simulink model "ros2webots_go_to_point_controller_model_cg"  (R2023a)
settings: Solver=FixedStepDiscrete  StartTime=0.0  StopTime=inf  FixedStep=0.05  RelTol=1e-3  EnableMultiTasking=on
model workspace (MAT data in the model file):
  Logfile_Data_Object = robotics.ros.BagSelection
  Logfile_Data_Object.FilePath = '\\wsl.localhost\ubuntu\home\mjavadzallaghi\ros2_ws\ros2webots\baglog\rosbot_data_20240125_225927.bag'
  Logfile_Data_Object.StartTime = 1706210981.23
  Logfile_Data_Object.EndTime = 1706211126.25
  Logfile_Data_Object.NumMessages = 508
  Logfile_Data_Object.AvailableTopics = table
  Logfile_Data_Object.AvailableTopics.data{1} = [73; 435]
  Logfile_Data_Object.AvailableTopics.data{2} = categorical
  Logfile_Data_Object.AvailableTopics.data{2}.categoryNames = {'geometry_msgs/Twist'; 'sensor_msgs/Imu'}
  Logfile_Data_Object.AvailableTopics.data{2}.codes = [1; 2]
  Logfile_Data_Object.AvailableTopics.data{3}{1} = 'geometry_msgs/Vector3 Linear
    |   double X
    |   double Y
    |   double Z
    | geometry_msgs/Vector3 Angular
    |   double X
    |   double Y
    |   double Z
    | '
  Logfile_Data_Object.AvailableTopics.data{3}{2} = 'std_msgs/Header Header
    |   uint32 Seq
    |   Time Stamp
    |   char FrameId
    | geometry_msgs/Quaternion Orientation
    |   double X
    |   double Y
    |   double Z
    |   double W
    | double[9] OrientationCovariance
    | geometry_msgs/Vector3 AngularVelocity
    |   double X
    |   double Y
    |   double Z
    | double[9] AngularVelocityCovariance
    | geometry_msgs/Vector3 LinearAcceleration
    |   double X
    |   double Y
    |   double Z
    | double[9] LinearAccelerationCovariance
    | '
  Logfile_Data_Object.AvailableTopics.ndims = 2
  Logfile_Data_Object.AvailableTopics.nrows = 2
  Logfile_Data_Object.AvailableTopics.rownames = {'/webots/rosbot/command_vel'; '/webots/rosbot/imu'}
  Logfile_Data_Object.AvailableTopics.nvars = 3
  Logfile_Data_Object.AvailableTopics.varnames = {'NumMessages', 'MessageType', 'MessageDefinition'}
  Logfile_Data_Object.AvailableTopics.props.useVariableNamesOriginal = 0
  Logfile_Data_Object.AvailableTopics.props.useDimensionNamesOriginal = 0
  Logfile_Data_Object.AvailableTopics.props.CustomProps = struct()
  Logfile_Data_Object.AvailableTopics.props.VariableCustomProps = struct()
  Logfile_Data_Object.AvailableTopics.props.versionSavedFrom = 4
  Logfile_Data_Object.AvailableTopics.props.minCompatibleVersion = 1
  Logfile_Data_Object.AvailableTopics.props.incompatibilityMsg = ''
  Logfile_Data_Object.AvailableTopics.props.VersionSavedFrom = 4
  Logfile_Data_Object.AvailableTopics.props.Description = ''
  Logfile_Data_Object.AvailableTopics.props.VariableNamesOriginal = {}
  Logfile_Data_Object.AvailableTopics.props.DimensionNames = {'Row', 'Variables'}
  Logfile_Data_Object.AvailableTopics.props.DimensionNamesOriginal = {}
  Logfile_Data_Object.AvailableTopics.props.UserData = []
  Logfile_Data_Object.AvailableTopics.props.VariableDescriptions = {}
  Logfile_Data_Object.AvailableTopics.props.VariableUnits = {}
  Logfile_Data_Object.AvailableTopics.props.VariableContinuity = {}
  Logfile_Data_Object.MessageList = table
  Logfile_Data_Object.MessageList.data{1} = [1706210981.23 1706210981.23 1706210981.23 1706210983.05 1706210983.38 1706210983.7 1706210984.04 1706210984.38 1706210984.72 1706210985.07 1706210985.41 1706210985.73 ... (508 elements, 508x1)]
  Logfile_Data_Object.MessageList.data{2} = categorical
  Logfile_Data_Object.MessageList.data{2}.categoryNames = {'/webots/rosbot/command_vel'; '/webots/rosbot/imu'}
  Logfile_Data_Object.MessageList.data{2}.codes = [1; 1; 1; 2; 2; 2; 2; 2; 2; 2; 2; 1; 1; 1; 2; 2; 2; 2; 2; 2; 2; 2; 2; 2; 2; 2; 2; 2; 2; 2; 2; 2; 2; 2; 2; 2; 2; 2; 1; 1; 1; 2; 2; 2; 2; 2; 2; 2; 2; 2; 2; 2; 2; 2; 2; 2; 2; 2; 2; 2; 2; 2; 2; 2; 2; 2; 2; 1; 1; 1; 2; 2; 2; 2; 2; 2; 2; 2; 2; 2; 2; 2; 2; 2; 2; 2; 2; 2; 2; 2; 2; 1; 1; 1; 2; 2; 2; 2; 2; 2; 2; 2; 2; 2; 2; 2; 2; 2; 2; 2; 2; 2; 2; 2; 2; 2; 2; 2; 1; 1; 2; 1; 2; 2; 2; 2; 2; 2; 2; 2; 2; 2; 2; 2; 2; 2; 2; 2; 2; 2; 2; 2; 2; 2; 2; 2; 2; 2; 2; 2; 2; 2; 2; 2; 2; 2; 2; 2; 2; 2; 2; 2; 2; 2; 2; 2; 1; 1; 1; 2; 2; 2; 2; 2; 2; 2; 2; 2; 2; 2; 2; 2; 2; 2; 2; 2; 2; 2; 2; 2; 2; 2; 2; 1; 1; 1; 2; 2; 2; 2; 2; 2; 2; 2; 2; 2; 2; 2; 2; 2; 2; 2; 2; 2; 2; 2; 2; 2; 2; 2; 2; 2; 2; 1; 1; 1; 2; 2; 2; 2; 2; 2; 2; 2; 2; 2; 2; 2; 2; 2; 2; 2; 2; 2; 2; 2; 2; 2; 2; 2; 2; 2; 1; 1; 1; 2; 2; 2; 2; 2; 2; 2; 2; 2; 2; 2; 2; 2; 2; 2; 2; 2; 2; 2; 2; 1; 1; 1; 2; 2; 2; 2; 2; 2; 2; 2; 2; 2; 2; 2; 2; 2; 2; 2; 2; 2; 2; 2; 2; 2; 2; 2; 2; 1; 1; 1; 2; 2; 2; 2; 2; 2; 2; 1; 1; 2; 1; 2; 2; 2; 2; 2; 2; 1; 1; 1; 2; 2; 2; 2; 2; 2; 2; 2; 2; 2; 2; 2; 1; 1; 1; 2; 2; 2; 2; 2; 2; 2; 2; 2; 2; 2; 2; 2; 2; 2; 2; 2; 2; 2; 1; 1; 1; 2; 2; 2; 2; 2; 2; 2; 2; 2; 1; 1; 1; 2; 2; 2; 2; 2; 2; 2; 2; 2; 2; 2; 2; 1; 1; 1; 2; 2; 2; 2; 2; 2; 1; 1; 1; 2; 2; 2; 2; 2; 2; 2; 2; 2; 2; 2; 2; 1; 1; 1; 2; 2; 2; 2; 2; 2; 2; 2; 2; 2; 1; 1; 1; 2; 2; 2; 2; 2; 2; 2; 2; 2; 2; 1; 1; 1; 2; 2; 2; 2; 2; 2; 2; 1; 1; 1; 2; 2; 2; 2; 2; 2; 2; 2; 2; 2; 2; 2; 2; 2; 2; 2; 1; 1; 1; 2; 2; 2; 2; 2; 2; 2; 2; 2; 2; 2; 2; 2; 2; 2; 2; 1; 2; 2; 2; 2; 2; 2; 2; 2; 2; 2; 2; 2; 2; 2; 2; 2; 2; 2; 2; 2; 2; 2]
  Logfile_Data_Object.MessageList.data{3} = categorical
  Logfile_Data_Object.MessageList.data{3}.categoryNames = {'geometry_msgs/Twist'; 'sensor_msgs/Imu'}
  Logfile_Data_Object.MessageList.data{3}.codes = [1; 1; 1; 2; 2; 2; 2; 2; 2; 2; 2; 1; 1; 1; 2; 2; 2; 2; 2; 2; 2; 2; 2; 2; 2; 2; 2; 2; 2; 2; 2; 2; 2; 2; 2; 2; 2; 2; 1; 1; 1; 2; 2; 2; 2; 2; 2; 2; 2; 2; 2; 2; 2; 2; 2; 2; 2; 2; 2; 2; 2; 2; 2; 2; 2; 2; 2; 1; 1; 1; 2; 2; 2; 2; 2; 2; 2; 2; 2; 2; 2; 2; 2; 2; 2; 2; 2; 2; 2; 2; 2; 1; 1; 1; 2; 2; 2; 2; 2; 2; 2; 2; 2; 2; 2; 2; 2; 2; 2; 2; 2; 2; 2; 2; 2; 2; 2; 2; 1; 1; 2; 1; 2; 2; 2; 2; 2; 2; 2; 2; 2; 2; 2; 2; 2; 2; 2; 2; 2; 2; 2; 2; 2; 2; 2; 2; 2; 2; 2; 2; 2; 2; 2; 2; 2; 2; 2; 2; 2; 2; 2; 2; 2; 2; 2; 2; 1; 1; 1; 2; 2; 2; 2; 2; 2; 2; 2; 2; 2; 2; 2; 2; 2; 2; 2; 2; 2; 2; 2; 2; 2; 2; 2; 1; 1; 1; 2; 2; 2; 2; 2; 2; 2; 2; 2; 2; 2; 2; 2; 2; 2; 2; 2; 2; 2; 2; 2; 2; 2; 2; 2; 2; 2; 1; 1; 1; 2; 2; 2; 2; 2; 2; 2; 2; 2; 2; 2; 2; 2; 2; 2; 2; 2; 2; 2; 2; 2; 2; 2; 2; 2; 2; 1; 1; 1; 2; 2; 2; 2; 2; 2; 2; 2; 2; 2; 2; 2; 2; 2; 2; 2; 2; 2; 2; 2; 1; 1; 1; 2; 2; 2; 2; 2; 2; 2; 2; 2; 2; 2; 2; 2; 2; 2; 2; 2; 2; 2; 2; 2; 2; 2; 2; 2; 1; 1; 1; 2; 2; 2; 2; 2; 2; 2; 1; 1; 2; 1; 2; 2; 2; 2; 2; 2; 1; 1; 1; 2; 2; 2; 2; 2; 2; 2; 2; 2; 2; 2; 2; 1; 1; 1; 2; 2; 2; 2; 2; 2; 2; 2; 2; 2; 2; 2; 2; 2; 2; 2; 2; 2; 2; 1; 1; 1; 2; 2; 2; 2; 2; 2; 2; 2; 2; 1; 1; 1; 2; 2; 2; 2; 2; 2; 2; 2; 2; 2; 2; 2; 1; 1; 1; 2; 2; 2; 2; 2; 2; 1; 1; 1; 2; 2; 2; 2; 2; 2; 2; 2; 2; 2; 2; 2; 1; 1; 1; 2; 2; 2; 2; 2; 2; 2; 2; 2; 2; 1; 1; 1; 2; 2; 2; 2; 2; 2; 2; 2; 2; 2; 1; 1; 1; 2; 2; 2; 2; 2; 2; 2; 1; 1; 1; 2; 2; 2; 2; 2; 2; 2; 2; 2; 2; 2; 2; 2; 2; 2; 2; 1; 1; 1; 2; 2; 2; 2; 2; 2; 2; 2; 2; 2; 2; 2; 2; 2; 2; 2; 1; 2; 2; 2; 2; 2; 2; 2; 2; 2; 2; 2; 2; 2; 2; 2; 2; 2; 2; 2; 2; 2; 2]
  Logfile_Data_Object.MessageList.data{4} = [5438 5532 5626 5720 6078 6436 6794 7152 7510 7868 8226 8584 ... (508 elements, 508x1)]
  Logfile_Data_Object.MessageList.ndims = 2
  Logfile_Data_Object.MessageList.nrows = 508
  Logfile_Data_Object.MessageList.nvars = 4
  Logfile_Data_Object.MessageList.varnames = {'Time', 'Topic', 'MessageType', 'FileOffset'}
  Logfile_Data_Object.MessageList.props.useVariableNamesOriginal = 0
  Logfile_Data_Object.MessageList.props.useDimensionNamesOriginal = 0
  Logfile_Data_Object.MessageList.props.CustomProps = struct()
  Logfile_Data_Object.MessageList.props.VariableCustomProps = struct()
  Logfile_Data_Object.MessageList.props.versionSavedFrom = 4
  Logfile_Data_Object.MessageList.props.minCompatibleVersion = 1
  Logfile_Data_Object.MessageList.props.incompatibilityMsg = ''
  Logfile_Data_Object.MessageList.props.VersionSavedFrom = 4
  Logfile_Data_Object.MessageList.props.Description = ''
  Logfile_Data_Object.MessageList.props.VariableNamesOriginal = {}
  Logfile_Data_Object.MessageList.props.DimensionNames = {'Row', 'Variables'}
  Logfile_Data_Object.MessageList.props.DimensionNamesOriginal = {}
  Logfile_Data_Object.MessageList.props.UserData = []
  Logfile_Data_Object.MessageList.props.VariableDescriptions = {}
  Logfile_Data_Object.MessageList.props.VariableUnits = {}
  Logfile_Data_Object.MessageList.props.VariableContinuity = {}
  Logfile_Data_Object.RawMessageBuffer = containers.Map
  Logfile_Data_Object.RawMessageBuffer.serialization.keys = {}
  Logfile_Data_Object.RawMessageBuffer.serialization.values = {}
  Logfile_Data_Object.RawMessageBuffer.serialization.uniformity = 0
  Logfile_Data_Object.RawMessageBuffer.serialization.keyType = 'char'
  Logfile_Data_Object.RawMessageBuffer.serialization.valueType = 'any'
  Logfile_Data_Object.ImgMessageBuffer = containers.Map
  Logfile_Data_Object.ImgMessageBuffer.serialization.keys = {}
  Logfile_Data_Object.ImgMessageBuffer.serialization.values = {}
  Logfile_Data_Object.ImgMessageBuffer.serialization.uniformity = 0
  Logfile_Data_Object.ImgMessageBuffer.serialization.keyType = 'char'
  Logfile_Data_Object.ImgMessageBuffer.serialization.valueType = 'any'
  Logfile_Data_Object.PointCloudBuffer = containers.Map
  Logfile_Data_Object.PointCloudBuffer.serialization.keys = {}
  Logfile_Data_Object.PointCloudBuffer.serialization.values = {}
  Logfile_Data_Object.PointCloudBuffer.serialization.uniformity = 0
  Logfile_Data_Object.PointCloudBuffer.serialization.keyType = 'char'
  Logfile_Data_Object.PointCloudBuffer.serialization.valueType = 'any'
  Logfile_Data_Object.LaserScanBuffer = containers.Map
  Logfile_Data_Object.LaserScanBuffer.serialization.keys = {}
  Logfile_Data_Object.LaserScanBuffer.serialization.values = {}
  Logfile_Data_Object.LaserScanBuffer.serialization.uniformity = 0
  Logfile_Data_Object.LaserScanBuffer.serialization.keyType = 'char'
  Logfile_Data_Object.LaserScanBuffer.serialization.valueType = 'any'
  Logfile_Data_Object.TopicTypeMap = containers.Map
  Logfile_Data_Object.TopicTypeMap.serialization.keys = {'/webots/rosbot/command_vel', '/webots/rosbot/imu'}
  Logfile_Data_Object.TopicTypeMap.serialization.values = {'geometry_msgs/Twist', 'sensor_msgs/Imu'}
  Logfile_Data_Object.TopicTypeMap.serialization.uniformity = 1
  Logfile_Data_Object.TopicTypeMap.serialization.keyType = 'char'
  Logfile_Data_Object.TopicTypeMap.serialization.valueType = 'char'
  Logfile_Data_Object.TopicDefinitionMap = containers.Map
  Logfile_Data_Object.TopicDefinitionMap.serialization.keys = {'/webots/rosbot/command_vel', '/webots/rosbot/imu'}
  Logfile_Data_Object.TopicDefinitionMap.serialization.values{1} = 'geometry_msgs/Vector3 Linear
    |   double X
    |   double Y
    |   double Z
    | geometry_msgs/Vector3 Angular
    |   double X
    |   double Y
    |   double Z
    | '
  Logfile_Data_Object.TopicDefinitionMap.serialization.values{2} = 'std_msgs/Header Header
    |   uint32 Seq
    |   Time Stamp
    |   char FrameId
    | geometry_msgs/Quaternion Orientation
    |   double X
    |   double Y
    |   double Z
    |   double W
    | double[9] OrientationCovariance
    | geometry_msgs/Vector3 AngularVelocity
    |   double X
    |   double Y
    |   double Z
    | double[9] AngularVelocityCovariance
    | geometry_msgs/Vector3 LinearAcceleration
    |   double X
    |   double Y
    |   double Z
    | double[9] LinearAccelerationCovariance
    | '
  Logfile_Data_Object.TopicDefinitionMap.serialization.uniformity = 1
  Logfile_Data_Object.TopicDefinitionMap.serialization.keyType = 'char'
  Logfile_Data_Object.TopicDefinitionMap.serialization.valueType = 'char'
  Logfile_Data_Object.messageTypeMap = containers.Map
  Logfile_Data_Object.messageTypeMap.serialization.keys = {}
  Logfile_Data_Object.messageTypeMap.serialization.values = {}
  Logfile_Data_Object.messageTypeMap.serialization.uniformity = 0
  Logfile_Data_Object.messageTypeMap.serialization.keyType = 'char'
  Logfile_Data_Object.messageTypeMap.serialization.valueType = 'any'
  Logfile_Data_Object.Parser = robotics.ros.internal.tf.TransformationTreeParser
  Logfile_Data_Object.Parser.UseObjectMsg = 1
  Logfile_Path = '\\wsl.localhost\ubuntu\home\mjavadzallaghi\ros2_ws\ros2webots\baglog\rosbot_data_20240125_225927.bag'
  Logfile_Playback_Duration = nan
  Logfile_Playback_Offset = nan
values from neighbouring files (symbols this model uses):
  laterl_PID_kd = 0.0    [ros2webots_go_to_point_controller_model_cg.sldd]
  laterl_PID_ki = 0.2    [ros2webots_go_to_point_controller_model_cg.sldd]
  laterl_PID_kp = 1.0    [ros2webots_go_to_point_controller_model_cg.sldd]
  longitudinal_speed_gain = 0.2    [ros2webots_go_to_point_controller_model_cg.sldd]
libraries: slpidlib x2, robotmobilelib x1, SignalEditorBlockLib x1
settings Model: DataDictionary=ros2webots_go_to_point_controller_model_cg.sldd  Creator=MJava  LastModifiedBy=MJava
settings SolverCC: AllowMultiTaskInputOutput=on  AutoInsertRateTranBlk=on
settings OptimizationCC: DefaultParameterBehavior=Inlined  EnhancedBackFolding=on  PassReuseOutputArgsAs=Individual arguments  ZeroExternalMemoryAtStartup=off  ZeroInternalMemoryAtStartup=off  MaxStackSize=64  OptimizeBlockOrder=speed  DifferentSizesBufferReuse=on  OptimizationCustomize=off  EfficientTunableParamExpr=on
settings DebuggingCC: ParameterTunabilityLossMsg=error
settings SFSimCC: MATLABDynamicMemAlloc=off  SimTargetLang=C++
settings RTWCC: Description=Embedded Coder  SystemTargetFile=ert.tlc  TemplateMakefile=ert_default_tmf  GenerateReport=on  Toolchain=Microsoft Visual C++ 2019 v16.0 | nmake (64-bit Windows)  BuildConfiguration=Faster Runs  LaunchReport=on  TargetLang=C++  GenerateWebview=on  GenerateCodeMetricsReport=on  CheckMdlBeforeBuild=Warning
settings CodeAppCC: ForceParamTrailComments=on  IgnoreCustomStorageClasses=off  OperatorAnnotations=on  SimulinkDataObjDesc=on  SFDataObjDesc=on  InsertBlockDesc=on
settings ERTTargetCC: TargetLangStandard=C++11 (ISO)  CodeInterfacePackaging=C++ class  RootIOFormat=Structure reference  ERTCustomFileTemplate=example_file_process.tlc

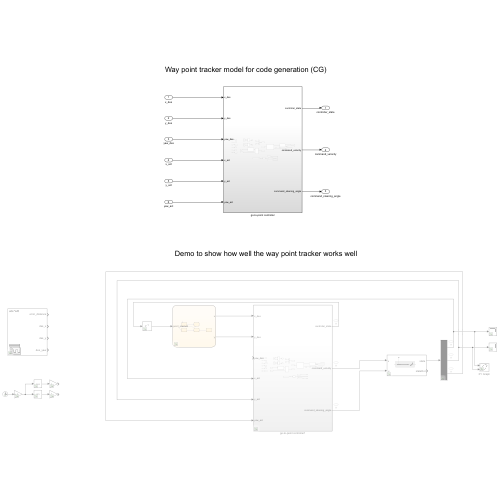
[thumbnail: Simulink's stored preview of the top-level diagram]
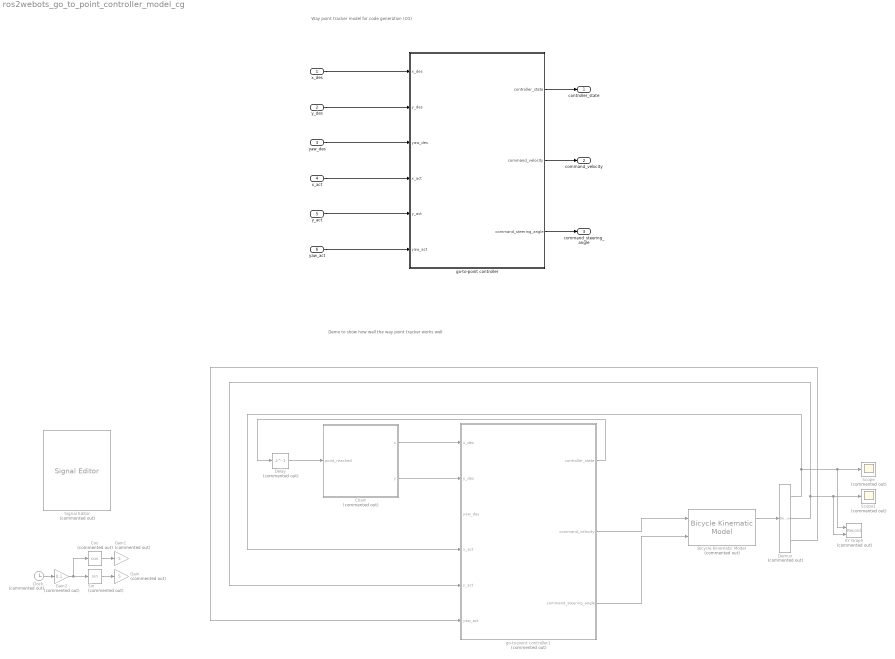
== system ros2webots_go_to_point_controller_model_cg ==
  note: Demo to show how well the way point tracker works well
  note: Way point tracker model for code generation (CG)
  x_des : Inport  OutDataTypeStr=double  PortDimensions=1
  y_des : Inport  Port=2
  yaw_des : Inport  Port=3
  x_act : Inport  Port=4
  y_act : Inport  Port=5
  yaw_act : Inport  Port=6
  Bicycle Kinematic Model : robotmobilelib/Bicycle Kinematic Model  Commented=on  VehicleInputs=Vehicle Speed & Steering Angle  WheelBase=0.2  VehicleSpeedRange=[-inf inf]  MaxSteeringAngle=pi/4  InitialState=[0; 0; 0]  SimulateUsing=Interpreted execution
  Chart : Stateflow chart  Commented=on  TreatAsAtomicUnit=on
  Clock : Clock  Commented=on
  Cos : Trigonometry  Commented=on  Operator=cos
  Delay : Delay  Commented=on  DelayLength=1  InitialCondition=1
  Demux : Demux  Commented=on  Outputs=3
  Gain : Gain  Commented=on  Gain=5
  Gain1 : Gain  Commented=on  Gain=5
  Gain2 : Gain  Commented=on  Gain=0.1
  Scope : Scope  Commented=on
  Scope1 : Scope  Commented=on
  Signal Editor : SignalEditorBlockLib/Signal Editor  Commented=on  FileName=controller_way_point_state_flow_test_scenario.mat  ActiveScenario=Scenario  ActiveSignal=error_distance  IsBus=off  OutputBusObjectStr=Bus: BusObject  SampleTime=0.05  Interpolate=off  ZeroCross=off  OutputAfterFinalValue=Setting to zero  Unit=inherit  PreserveSignalName=on  ApplySigPropsToAllScenarios=on
  Sin : Trigonometry  Commented=on
  XY Graph : Record  Commented=on  FileSettingsInternal="{\"entries\":[{\"content\":{\"excelSettings\":{\"content\":{},\"type\":\"Streamout.ExcelSettings\"}},\"type\":\"Streamout.FileSettingStorage\",\"uuid\":\"b027da48-4c5f-40c1-b71a-aa0128182c7a\"}],\"packageUris\":[\"http://schema.mathworks.com/mf0/streamout_blocks/R2020a\"],\"version\":\"1.0\"}"  Layout=[1 1]  SignalsInternal="{\"entries\":[{\"content\":{},\"type\":\"RecordBlkView.InputSignals\",\"uuid\":\"f54d1e1f-9c18-4039-bd87-6a5f989906ef\"}],\"packageUris\":[\"http://schema.mathworks.com/mf0/streamout_blocks/R2020a\"],\"version\":\"1.0\"}"  VisualizationBindings="{\"xyplotplugin\":{\"info\":[{\"series\":[],\"subplotID\":1}]}}"  CompatibilityTag=XY
  go-to-point controller : Subsystem
  go-to-point controller1 : Subsystem  Commented=on
  controller_state : Outport  PortDimensions=1
  command_velocity : Outport  Port=2  PortDimensions=1
  command_steering_angle : Outport  Port=3  PortDimensions=1
  wires:
  x_des/1 -> go-to-point controller/1(x_des)
  go-to-point controller/1(controller_state) -> controller_state/1
  y_des/1 -> go-to-point controller/2(y_des)
  y_act/1 -> go-to-point controller/5(y_act)
  x_act/1 -> go-to-point controller/4(x_act)
  yaw_des/1 -> go-to-point controller/3(yaw_des)
  yaw_act/1 -> go-to-point controller/6(yaw_act)
  go-to-point controller/2(command_velocity) -> command_velocity/1
  go-to-point controller/3(command_steering_angle) -> command_steering_angle/1
  Bicycle Kinematic Model/1 -> Demux/1
  Demux/1 -> go-to-point controller1/4(x_act), XY Graph/1, Scope/1
  Demux/2 -> go-to-point controller1/5(y_act), XY Graph/2, Scope1/1
  Demux/3 -> go-to-point controller1/6(yaw_act)
  go-to-point controller1/2(command_velocity) -> Bicycle Kinematic Model/1
  go-to-point controller1/3(command_steering_angle) -> Bicycle Kinematic Model/2
  go-to-point controller1/1(controller_state) -> Delay/1
  Delay/1 -> Chart/1(point_reached)
  Clock/1 -> Gain2/1
  Gain2/1 -> Cos/1, Sin/1
  Cos/1 -> Gain1/1
  Sin/1 -> Gain/1
  Chart/1(x) -> go-to-point controller1/1(x_des)
  Chart/2(y) -> go-to-point controller1/2(y_des)

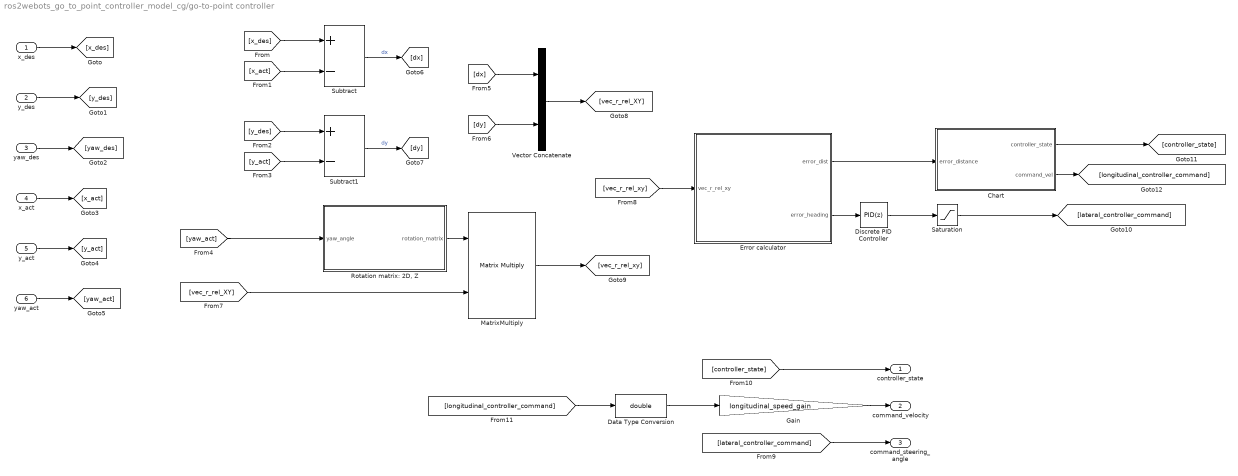
== system ros2webots_go_to_point_controller_model_cg/go-to-point controller ==
  x_des : Inport  OutDataTypeStr=double  PortDimensions=1
  y_des : Inport  Port=2  OutDataTypeStr=double  PortDimensions=1
  yaw_des : Inport  Port=3  OutDataTypeStr=double  PortDimensions=1
  x_act : Inport  Port=4  OutDataTypeStr=double  PortDimensions=1
  y_act : Inport  Port=5  OutDataTypeStr=double  PortDimensions=1
  yaw_act : Inport  Port=6  OutDataTypeStr=double  PortDimensions=1
  Chart : Stateflow chart  TreatAsAtomicUnit=on
  Data Type Conversion : DataTypeConversion  OutDataTypeStr=double  SaturateOnIntegerOverflow=off  RndMeth=Floor
  Discrete PID Controller : slpidlib/PID Controller  Controller=PID  Form=Parallel  TimeDomain=Discrete-time  UseExternalTs=off  SampleTime=-1  IntegratorMethod=Forward Euler  FilterMethod=Forward Euler  ControllerParametersSource=internal  P=laterl_PID_kp  I=laterl_PID_ki  UseKiTs=off  D=laterl_PID_kd  N=100  UseFilter=on  TunerSelectOption=Transfer Function Based (PID Tuner App)  InitialConditionSource=internal  InitialConditionForIntegrator=0  InitialConditionForFilter=0  DifferentiatorICPrevScaledInput=0  ExternalReset=none  TrackingMode=off  Kt=1  LimitOutput=off  SatLimitsSource=internal  UpperSaturationLimit=inf  LowerSaturationLimit=-inf  LinearizeAsGain=off  AntiWindupMode=none  Kb=1  LimitIntegrator=off  UpperIntegratorSaturationLimit=inf  LowerIntegratorSaturationLimit=-inf  POutMin=[]  POutMax=[]  IOutMin=[]  IOutMax=[]  DOutMin=[]  DOutMax=[]  NOutMin=[]  NOutMax=[]  SumOutMin=[]  SumOutMax=[]  SaturationOutMin=[]  SaturationOutMax=[]  PParamMin=[]  PParamMax=[]  IParamMin=[]  IParamMax=[]  DParamMin=[]  DParamMax=[]  NParamMin=[]  NParamMax=[]  KbParamMin=[]  KbParamMax=[]  KtParamMin=[]  KtParamMax=[]  KbOutMin=[]  KbOutMax=[]  KtOutMin=[]  KtOutMax=[]  IntegratorOutMin=[]  IntegratorOutMax=[]  FilterOutMin=[]  FilterOutMax=[]  SumI1OutMin=[]  SumI1OutMax=[]  SumI2OutMin=[]  SumI2OutMax=[]  SumI3OutMin=[]  SumI3OutMax=[]  SumI4OutMin=[]  SumI4OutMax=[]  SumDOutMin=[]  SumDOutMax=[]  DifferentiatorOutMin=[]  DifferentiatorOutMax=[]  FilterDiffOutCoefMin=[]  FilterDiffOutCoefMax=[]  ReciprocalOutMin=[]  ReciprocalOutMax=[]  SumDenOutMin=[]  SumDenOutMax=[]  SumNumOutMin=[]  SumNumOutMax=[]  DivideOutMin=[]  DivideOutMax=[]  UdiffTsProdOutMin=[]  UdiffTsProdOutMax=[]  NTsProdOutMin=[]  NTsProdOutMax=[]  UintegralTsProdOutMin=[]  UintegralTsProdOutMax=[]  UngainTsProdOutMin=[]  UngainTsProdOutMax=[]  ClampingZeroOutDataTypeStr=Inherit: Inherit via back propagation  ClampingZeroOutMin=[]  ClampingZeroOutMax=[]  FilterDenConstantOutDataTypeStr=Inherit: Inherit via back propagation  FilterDenConstantOutMin=[]  FilterDenConstantOutMax=[]  PCopyOutDataTypeStr=Inherit: Inherit via back propagation  PCopyOutMin=[]  PCopyOutMax=[]  NCopyOutDataTypeStr=Inherit: Inherit via back propagation  NCopyOutMin=[]  NCopyOutMax=[]  IntegratorContinuousStateAttributes=''  IntegratorStateMustResolveToSignalObject=off  IntegratorRTWStateStorageClass=Auto  FilterContinuousStateAttributes=''  FilterStateMustResolveToSignalObject=off  FilterRTWStateStorageClass=Auto  ParallelPVariant=InternalParameters  IdealPVariant=Disabled  IVariant=InternalParameters  DVariant=InternalParameters  IntegratorVariant=Discrete  SatVariant=Disabled  AWVariant=Passthrough  PCopyVariant=Disabled  TRVariant=Disabled  FdbkBlocksVariant=Forward  IdealPFdbkVariant=Disabled  SatFdbkVariant=Disabled  DerivativeFilterVariant=ForwardEulerFilter  NVariant=InternalParameters  NCopyVariant=Disabled  FilterICVariant=InternalICsFilter  IntegratorICVariant=InternalICs  ExternalResetVariant=Disabled  TRSumVariant=Passthrough  SumFdbkVariant=Disabled  SumVariant=Sum_PID  TsampFilterVariant=InternalTs  TsampNgainVariant=Passthrough  TsampIntegralVariant=Disabled_SignalSpec  ExternalSaturationOutDataTypeStr=Inherit: Same as second input
      settings: LibrarySourceBlock=simulink/Discrete/Discrete PID Controller
  Error calculator : MATLAB Function  TreatAsAtomicUnit=on
  Gain : Gain  Gain=longitudinal_speed_gain
  MatrixMultiply : Product  Multiplication=Matrix(*)
  "Rotation matrix: 2D, Z" : MATLAB Function  TreatAsAtomicUnit=on
  Saturation : Saturate  UpperLimit=pi/4  LowerLimit=-pi/4
  Subtract : Sum  Inputs=+-
  Subtract1 : Sum  Inputs=+-
  Vector Concatenate : Concatenate
  controller_state : Outport  OutDataTypeStr=uint8  PortDimensions=1
  command_velocity : Outport  Port=2  OutDataTypeStr=double  PortDimensions=1
  command_steering_angle : Outport  Port=3  OutDataTypeStr=double  PortDimensions=1
  wires:
  x_des/1 -> [x_des]
  y_des/1 -> [y_des]
  yaw_act/1 -> [yaw_act]
  y_act/1 -> [y_act]
  x_act/1 -> [x_act]
  yaw_des/1 -> [yaw_des]
  [x_des] -> Subtract/1
  [x_act] -> Subtract/2
  Subtract/1 -> [dx]  "dx"
  [y_act] -> Subtract1/2
  Subtract1/1 -> [dy]  "dy"
  [y_des] -> Subtract1/1
  "Rotation matrix: 2D, Z"/1(rotation_matrix) -> MatrixMultiply/1
  [yaw_act] -> "Rotation matrix: 2D, Z"/1(yaw_angle)
  [dx] -> Vector Concatenate/1
  [dy] -> Vector Concatenate/2
  Vector Concatenate/1 -> [vec_r_rel_XY]
  [vec_r_rel_XY] -> MatrixMultiply/2
  MatrixMultiply/1 -> [vec_r_rel_xy]
  [vec_r_rel_xy] -> Error calculator/1(vec_r_rel_xy)
  Error calculator/2(error_heading) -> Discrete PID Controller/1
  Discrete PID Controller/1 -> Saturation/1
  [lateral_controller_command] -> command_steering_angle/1
  Error calculator/1(error_dist) -> Chart/1(error_distance)
  Chart/1(controller_state) -> [controller_state]
  [controller_state] -> controller_state/1
  Chart/2(command_vel) -> [longitudinal_controller_command]
  [longitudinal_controller_command] -> Data Type Conversion/1
  Gain/1 -> command_velocity/1
  Data Type Conversion/1 -> Gain/1
  Saturation/1 -> [lateral_controller_command]

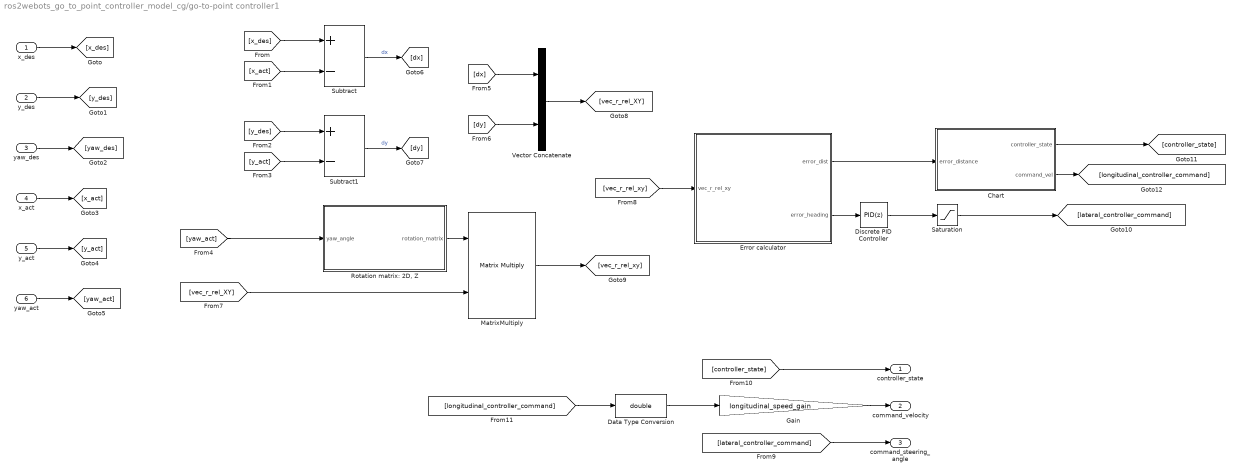
== system ros2webots_go_to_point_controller_model_cg/go-to-point controller1 ==
  x_des : Inport  OutDataTypeStr=double  PortDimensions=1
  y_des : Inport  Port=2  OutDataTypeStr=double  PortDimensions=1
  yaw_des : Inport  Port=3  OutDataTypeStr=double  PortDimensions=1
  x_act : Inport  Port=4  OutDataTypeStr=double  PortDimensions=1
  y_act : Inport  Port=5  OutDataTypeStr=double  PortDimensions=1
  yaw_act : Inport  Port=6  OutDataTypeStr=double  PortDimensions=1
  Chart : Stateflow chart  TreatAsAtomicUnit=on
  Data Type Conversion : DataTypeConversion  OutDataTypeStr=double  SaturateOnIntegerOverflow=off  RndMeth=Floor
  Discrete PID Controller : slpidlib/PID Controller  Controller=PID  Form=Parallel  TimeDomain=Discrete-time  UseExternalTs=off  SampleTime=-1  IntegratorMethod=Forward Euler  FilterMethod=Forward Euler  ControllerParametersSource=internal  P=laterl_PID_kp  I=laterl_PID_ki  UseKiTs=off  D=laterl_PID_kd  N=100  UseFilter=on  TunerSelectOption=Transfer Function Based (PID Tuner App)  InitialConditionSource=internal  InitialConditionForIntegrator=0  InitialConditionForFilter=0  DifferentiatorICPrevScaledInput=0  ExternalReset=none  TrackingMode=off  Kt=1  LimitOutput=off  SatLimitsSource=internal  UpperSaturationLimit=inf  LowerSaturationLimit=-inf  LinearizeAsGain=off  AntiWindupMode=none  Kb=1  LimitIntegrator=off  UpperIntegratorSaturationLimit=inf  LowerIntegratorSaturationLimit=-inf  POutMin=[]  POutMax=[]  IOutMin=[]  IOutMax=[]  DOutMin=[]  DOutMax=[]  NOutMin=[]  NOutMax=[]  SumOutMin=[]  SumOutMax=[]  SaturationOutMin=[]  SaturationOutMax=[]  PParamMin=[]  PParamMax=[]  IParamMin=[]  IParamMax=[]  DParamMin=[]  DParamMax=[]  NParamMin=[]  NParamMax=[]  KbParamMin=[]  KbParamMax=[]  KtParamMin=[]  KtParamMax=[]  KbOutMin=[]  KbOutMax=[]  KtOutMin=[]  KtOutMax=[]  IntegratorOutMin=[]  IntegratorOutMax=[]  FilterOutMin=[]  FilterOutMax=[]  SumI1OutMin=[]  SumI1OutMax=[]  SumI2OutMin=[]  SumI2OutMax=[]  SumI3OutMin=[]  SumI3OutMax=[]  SumI4OutMin=[]  SumI4OutMax=[]  SumDOutMin=[]  SumDOutMax=[]  DifferentiatorOutMin=[]  DifferentiatorOutMax=[]  FilterDiffOutCoefMin=[]  FilterDiffOutCoefMax=[]  ReciprocalOutMin=[]  ReciprocalOutMax=[]  SumDenOutMin=[]  SumDenOutMax=[]  SumNumOutMin=[]  SumNumOutMax=[]  DivideOutMin=[]  DivideOutMax=[]  UdiffTsProdOutMin=[]  UdiffTsProdOutMax=[]  NTsProdOutMin=[]  NTsProdOutMax=[]  UintegralTsProdOutMin=[]  UintegralTsProdOutMax=[]  UngainTsProdOutMin=[]  UngainTsProdOutMax=[]  ClampingZeroOutDataTypeStr=Inherit: Inherit via back propagation  ClampingZeroOutMin=[]  ClampingZeroOutMax=[]  FilterDenConstantOutDataTypeStr=Inherit: Inherit via back propagation  FilterDenConstantOutMin=[]  FilterDenConstantOutMax=[]  PCopyOutDataTypeStr=Inherit: Inherit via back propagation  PCopyOutMin=[]  PCopyOutMax=[]  NCopyOutDataTypeStr=Inherit: Inherit via back propagation  NCopyOutMin=[]  NCopyOutMax=[]  IntegratorContinuousStateAttributes=''  IntegratorStateMustResolveToSignalObject=off  IntegratorRTWStateStorageClass=Auto  FilterContinuousStateAttributes=''  FilterStateMustResolveToSignalObject=off  FilterRTWStateStorageClass=Auto  ParallelPVariant=InternalParameters  IdealPVariant=Disabled  IVariant=InternalParameters  DVariant=InternalParameters  IntegratorVariant=Discrete  SatVariant=Disabled  AWVariant=Passthrough  PCopyVariant=Disabled  TRVariant=Disabled  FdbkBlocksVariant=Forward  IdealPFdbkVariant=Disabled  SatFdbkVariant=Disabled  DerivativeFilterVariant=ForwardEulerFilter  NVariant=InternalParameters  NCopyVariant=Disabled  FilterICVariant=InternalICsFilter  IntegratorICVariant=InternalICs  ExternalResetVariant=Disabled  TRSumVariant=Passthrough  SumFdbkVariant=Disabled  SumVariant=Sum_PID  TsampFilterVariant=InternalTs  TsampNgainVariant=Passthrough  TsampIntegralVariant=Disabled_SignalSpec  ExternalSaturationOutDataTypeStr=Inherit: Same as second input
      settings: LibrarySourceBlock=simulink/Discrete/Discrete PID Controller
  Error calculator : MATLAB Function  TreatAsAtomicUnit=on
  Gain : Gain  Gain=longitudinal_speed_gain
  MatrixMultiply : Product  Multiplication=Matrix(*)
  "Rotation matrix: 2D, Z" : MATLAB Function  TreatAsAtomicUnit=on
  Saturation : Saturate  UpperLimit=pi/4  LowerLimit=-pi/4
  Subtract : Sum  Inputs=+-
  Subtract1 : Sum  Inputs=+-
  Vector Concatenate : Concatenate
  controller_state : Outport  OutDataTypeStr=uint8  PortDimensions=1
  command_velocity : Outport  Port=2  OutDataTypeStr=double  PortDimensions=1
  command_steering_angle : Outport  Port=3  OutDataTypeStr=double  PortDimensions=1
  wires:
  x_des/1 -> [x_des]
  y_des/1 -> [y_des]
  yaw_act/1 -> [yaw_act]
  y_act/1 -> [y_act]
  x_act/1 -> [x_act]
  yaw_des/1 -> [yaw_des]
  [x_des] -> Subtract/1
  [x_act] -> Subtract/2
  Subtract/1 -> [dx]  "dx"
  [y_act] -> Subtract1/2
  Subtract1/1 -> [dy]  "dy"
  [y_des] -> Subtract1/1
  "Rotation matrix: 2D, Z"/1(rotation_matrix) -> MatrixMultiply/1
  [yaw_act] -> "Rotation matrix: 2D, Z"/1(yaw_angle)
  [dx] -> Vector Concatenate/1
  [dy] -> Vector Concatenate/2
  Vector Concatenate/1 -> [vec_r_rel_XY]
  [vec_r_rel_XY] -> MatrixMultiply/2
  MatrixMultiply/1 -> [vec_r_rel_xy]
  [vec_r_rel_xy] -> Error calculator/1(vec_r_rel_xy)
  Error calculator/2(error_heading) -> Discrete PID Controller/1
  Discrete PID Controller/1 -> Saturation/1
  [lateral_controller_command] -> command_steering_angle/1
  Error calculator/1(error_dist) -> Chart/1(error_distance)
  Chart/1(controller_state) -> [controller_state]
  [controller_state] -> controller_state/1
  Chart/2(command_vel) -> [longitudinal_controller_command]
  [longitudinal_controller_command] -> Data Type Conversion/1
  Gain/1 -> command_velocity/1
  Data Type Conversion/1 -> Gain/1
  Saturation/1 -> [lateral_controller_command]

== stateflow chart ros2webots_go_to_point_controller_model_cg/go-to-point controller1/Chart ==
  state controller_off
    controller_state = 0;
    command_vel = 0;
  state controller_on
    controller_state = 1;
    command_vel = 1;
  (default) -> controller_off
  controller_off -> controller_on : [error_distance >=...
      | param_error_distance]
  controller_on -> controller_off : [error_distance <...
      | 1.05*param_error_distance]
  data: controller_state output uint8; error_distance input; param_error_distance constant double =0.20; command_vel output uint8

== matlab function ros2webots_go_to_point_controller_model_cg/go-to-point controller1/Error calculator ==
  data: vec_r_rel_xy input; error_dist output; error_heading output
function [error_dist, error_heading] = tracking_error(vec_r_rel_xy)

error_dist = sqrt(vec_r_rel_xy(1)^2 + vec_r_rel_xy(2)^2);
error_heading = atan2(vec_r_rel_xy(2), vec_r_rel_xy(1)); % <0 --> turns left, >0 --> turns right

== matlab function ros2webots_go_to_point_controller_model_cg/go-to-point controller1/Rotation matrix: 2D, Z ==
  data: yaw_angle input; rotation_matrix output
function rotation_matrix = rotate_2d_around_Z(yaw_angle)

r_11 = cos(yaw_angle);
r_12 = sin(yaw_angle);
r_21 = -sin(yaw_angle);
r_22 = cos(yaw_angle);

rotation_matrix = [r_11, r_12; r_21, r_22];

== stateflow chart ros2webots_go_to_point_controller_model_cg/Chart ==
  state p0
    x=5;
    y = 0;
  state p1
    x=5;
    y = 3;
  state p2
    x=-5;
    y = 3;
  state p3
    x=-5;
    y = 0;
  state p4
    x=0;
    y = 0;
  (default) -> p0
  p0 -> p1 : [point_reached==0]
  p1 -> p2 : [point_reached==0]
  p2 -> p3 : [point_reached==0]
  p3 -> p4 : [point_reached==0]
  data: x output; y output; point_reached input

== stateflow chart ros2webots_go_to_point_controller_model_cg/go-to-point controller/Chart ==
  state controller_off
    controller_state = 0;
    command_vel = 0;
  state controller_on
    controller_state = 1;
    command_vel = 1;
  (default) -> controller_off
  controller_off -> controller_on : [error_distance >=...
      | param_error_distance]
  controller_on -> controller_off : [error_distance <...
      | 1.05*param_error_distance]
  data: controller_state output uint8; error_distance input; param_error_distance constant double =0.20; command_vel output uint8

== matlab function ros2webots_go_to_point_controller_model_cg/go-to-point controller/Error calculator ==
  data: vec_r_rel_xy input; error_dist output; error_heading output
function [error_dist, error_heading] = tracking_error(vec_r_rel_xy)

error_dist = sqrt(vec_r_rel_xy(1)^2 + vec_r_rel_xy(2)^2);
error_heading = atan2(vec_r_rel_xy(2), vec_r_rel_xy(1)); % <0 --> turns left, >0 --> turns right

== matlab function ros2webots_go_to_point_controller_model_cg/go-to-point controller/Rotation matrix: 2D, Z ==
  data: yaw_angle input; rotation_matrix output
function rotation_matrix = rotate_2d_around_Z(yaw_angle)

r_11 = cos(yaw_angle);
r_12 = sin(yaw_angle);
r_21 = -sin(yaw_angle);
r_22 = cos(yaw_angle);

rotation_matrix = [r_11, r_12; r_21, r_22];
